simulink model "Switch"  (R2020a)
settings: Solver=VariableStepAuto  StartTime=0.0  StopTime=10.0  RelTol=1e-3
settings Model: Creator=royde  LastModifiedBy=royde

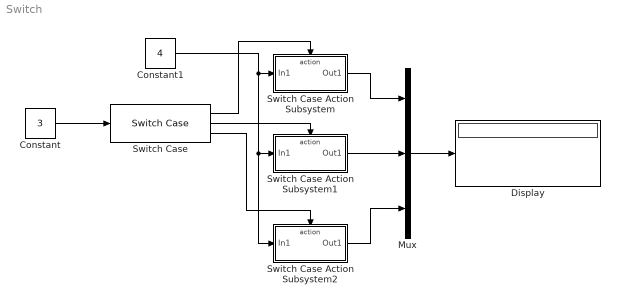
== system Switch ==
  Constant : Constant  Value=3
  Constant1 : Constant  Value=4
  Display : Display
  Mux : Mux  Inputs=3
  Switch Case : SwitchCase  CaseConditions={1,2}
  Switch Case Action Subsystem : Subsystem  TreatAsAtomicUnit=on
  Switch Case Action Subsystem1 : Subsystem  TreatAsAtomicUnit=on
  Switch Case Action Subsystem2 : Subsystem  TreatAsAtomicUnit=on
  wires:
  Switch Case/1 -> Switch Case Action Subsystem/Action
  Switch Case/2 -> Switch Case Action Subsystem1/Action
  Switch Case/3 -> Switch Case Action Subsystem2/Action
  Constant/1 -> Switch Case/1
  Mux/1 -> Display/1
  Switch Case Action Subsystem/1(Out1) -> Mux/1
  Switch Case Action Subsystem2/1(Out1) -> Mux/3
  Switch Case Action Subsystem1/1(Out1) -> Mux/2
  Constant1/1 -> Switch Case Action Subsystem2/1(In1), Switch Case Action Subsystem1/1(In1), Switch Case Action Subsystem/1(In1)

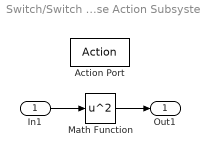
== system Switch/Switch Case Action Subsystem ==
  In1 : Inport
  Action Port : ActionPort  ActionPortLabel=case [ 1 ]:
  Math Function : Math  Operator=square  SaturateOnIntegerOverflow=on
  Out1 : Outport
  wires:
  In1/1 -> Math Function/1
  Math Function/1 -> Out1/1

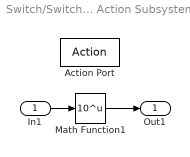
== system Switch/Switch Case Action Subsystem1 ==
  In1 : Inport
  Action Port : ActionPort  ActionPortLabel=case [ 2 ]:
  Math Function1 : Math  Operator=10^u  SaturateOnIntegerOverflow=on
  Out1 : Outport
  wires:
  Math Function1/1 -> Out1/1
  In1/1 -> Math Function1/1

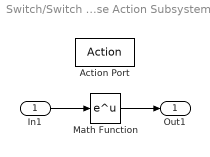
== system Switch/Switch Case Action Subsystem2 ==
  In1 : Inport
  Action Port : ActionPort  ActionPortLabel=default:
  Math Function : Math  SaturateOnIntegerOverflow=on
  Out1 : Outport
  wires:
  In1/1 -> Math Function/1
  Math Function/1 -> Out1/1
